simulink model "ulazna_f"  (Simulink 8.0)
settings: Solver=ode1  StartTime=0.0  StopTime=10.0  FixedStep=0.001  RelTol=1e-3
settings Model: Creator=Niko  LastModifiedBy=Niko

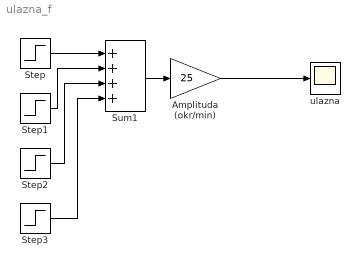
== system ulazna_f ==
  Amplituda (okr/min) : Gain  Gain=25
  Step : Step
  Step1 : Step  Time=2  After=-1
  Step2 : Step  Time=3  After=-1
  Step3 : Step  Time=4
  Sum1 : Sum  Inputs=++++
  ulazna : Scope
      settings: TimeRange=5  YMin=0  YMax=30  SaveName=ulazna_f  SampleInput=on
  wires:
  Sum1/1 -> Amplituda (okr/min)/1
  Step3/1 -> Sum1/4
  Step2/1 -> Sum1/3
  Step1/1 -> Sum1/2
  Step/1 -> Sum1/1
  Amplituda (okr/min)/1 -> ulazna/1
